simulink library "csu_ctp_coarse_thruster_pulse_command_new_lib"  (R2015b)
settings: Solver=ode113  StartTime=0.0  StopTime=10.0  RelTol=1e-3
values from neighbouring files (symbols this model uses):
  cac_acs_minimum_coarse_thruster_ontime = 30    [csc_cac_coarse_acs_ctrl_init.m]
  cac_acs_time_gain_x = 20.0    (= 20)    [csc_cac_coarse_acs_ctrl_init.m]
  cac_acs_time_gain_y = 20.0    (= 20)    [csc_cac_coarse_acs_ctrl_init.m]
  cac_acs_time_gain_z = 20.0    (= 20)    [csc_cac_coarse_acs_ctrl_init.m]
  cac_coarse_desired_thrust_gain = 1.0    (= 1)    [csc_cac_coarse_acs_ctrl_init.m]
  cac_coarse_thruster_force = psp_coarse_acs_thrust    [csc_cac_coarse_acs_ctrl_prep.m]
  cac_coarse_thruster_trq_x = cac_coarse_thruster_trq_x + cac_coarse_thruster_force*cac_coarse_trq_matx(cac_thruster_alloc_coarse_x_plus(i),1)    [csc_cac_coarse_acs_ctrl_prep.m]
  cac_coarse_thruster_trq_y = cac_coarse_thruster_trq_y + cac_coarse_thruster_force*cac_coarse_trq_matx(cac_thruster_alloc_coarse_y_plus(i),2)    [csc_cac_coarse_acs_ctrl_prep.m]
  cac_coarse_thruster_trq_z = cac_coarse_thruster_trq_z + cac_coarse_thruster_force*cac_coarse_trq_matx(cac_thruster_alloc_coarse_z_plus(i),3)    [csc_cac_coarse_acs_ctrl_prep.m]
  cac_max_thrust_to_weight_ratio = 1.05    [csc_cac_coarse_acs_ctrl_init.m]
  cac_saturation_axial_force = 0*cac_coarse_thruster_force*cosd(15)+4*cac_coarse_thruster_force    [csc_cac_coarse_acs_ctrl_prep.m]
  cac_total_trq_axial_force_matx = [cac_coarse_thruster_force*cac_coarse_trq_matx';cac_coarse_thruster_force_axial]    [csc_cac_coarse_acs_ctrl_prep.m]
undefined symbols (not defined in the file or in its folder): cac_num_variable, cac_thr_control, cac_thruster_alloc_pad_coarse_x_tq_full_on, cac_thruster_alloc_pad_coarse_x_tq_variable, cac_thruster_alloc_pad_coarse_y_tq_full_on, cac_thruster_alloc_pad_coarse_y_tq_variable, cac_trq_control, emp_initial_mass, gal_grav_surface_topo
libraries: simulink x12, util_info_lib x2
(part 1 of 2)
settings Model: Creator=Jim Kaidy  LastModifiedBy=jimkaidy
settings DataIOCC: SaveFormat=Array  SignalLoggingSaveFormat=ModelDataLogs
settings DebuggingCC: AlgebraicLoopMsg=error  ArtificialAlgebraicLoopMsg=error  UnderspecifiedInitializationDetection=Classic  MergeDetectMultiDrivingBlocksExec=none  SolverPrmCheckMsg=warning
settings HardwareCC: ProdBitPerPointer=32  ProdLargestAtomicFloat=None  ProdIntDivRoundTo=Undefined  ProdEndianess=Unspecified  ProdWordSize=32  ProdHWDeviceType=32-bit Generic
settings GRTTargetCC: GeneratePreprocessorConditionals=Disable all
settings ConfigComp: CovModelRefEnable=Off  CovSFcnEnable=off

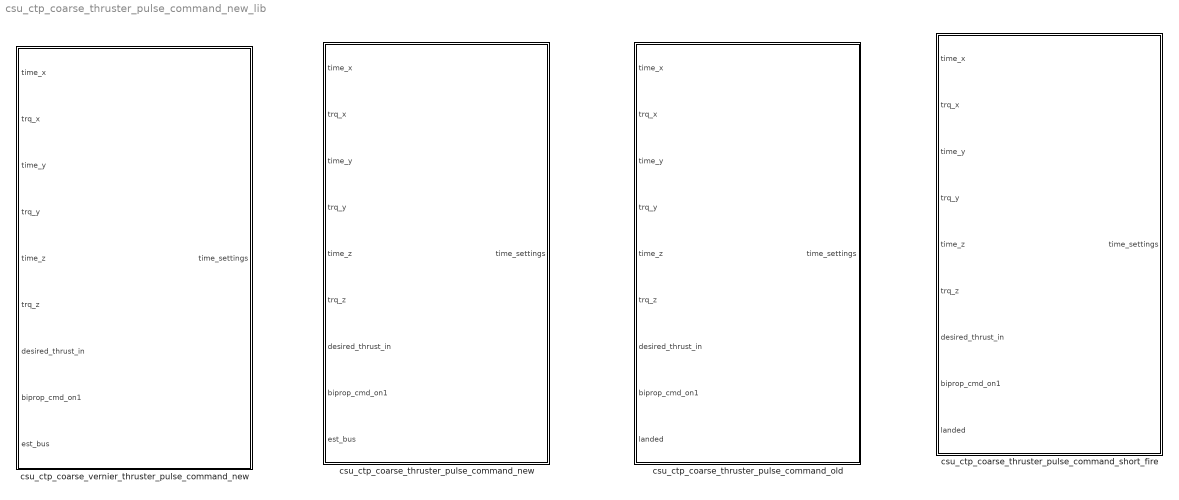
== system csu_ctp_coarse_thruster_pulse_command_new_lib ==
  csu_ctp_coarse_thruster_pulse_command_new : Subsystem
  csu_ctp_coarse_thruster_pulse_command_old : Subsystem
  csu_ctp_coarse_thruster_pulse_command_short_fire : Subsystem
  csu_ctp_coarse_vernier_thruster_pulse_command_new : Subsystem

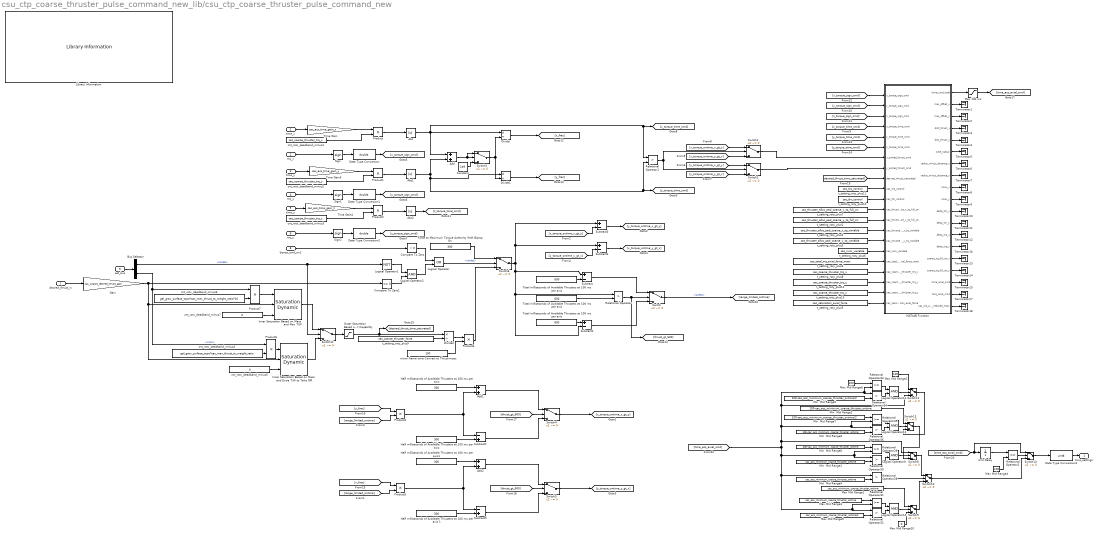
== system csu_ctp_coarse_thruster_pulse_command_new_lib/csu_ctp_coarse_thruster_pulse_command_new ==
  time_x : Inport
  "trq_x " : Inport  Port=2
  time_y : Inport  Port=3
  trq_y : Inport  Port=4
  time_z : Inport  Port=5
  trq_z : Inport  Port=6
  desired_thrust_in : Inport  Port=7
  biprop_cmd_on1 : Inport  Port=8
  est_bus : Inport  Port=9
  Abs : Abs
  Abs1 : Abs
  Abs2 : Abs
  Add : Sum
  Add1 : Sum
  Add2 : Sum
  Bus Selector : BusSelector  OutputSignals=landed,mass
  Compare To Zero : simulink/Logic and Bit Operations/Compare To Zero  relop=>  OutDataTypeStr=boolean
  Compare To Zero1 : simulink/Logic and Bit Operations/Compare To Zero  relop===  OutDataTypeStr=boolean
  Constant : Constant  Value=1e9
  Data Type Conversion : DataTypeConversion  OutDataTypeStr=double
  Data Type Conversion1 : DataTypeConversion  OutDataTypeStr=double
  Data Type Conversion2 : DataTypeConversion  OutDataTypeStr=double
  Data Type Conversion3 : DataTypeConversion  OutDataTypeStr=uint8
  Divide : Product  Inputs=*/
  Divide1 : Product  Inputs=*/
  Divide2 : Product  Inputs=*/
  Force to Maximum Torque Authority With Biprop On : Constant  Value=300
  Gain : Gain  Gain=cac_coarse_desired_thrust_gain
  Half milliseconds of Available Thrusters at 100 ms per axis : Constant  Value=300
  "Half milliseconds of Available Thrusters at 100 ms per axis " : Constant  Value=300
  Half milliseconds of Available Thrusters at 100 ms per axis 1 : Constant  Value=300
  Half milliseconds of Available Thrusters at 100 ms per axis1 : Constant  Value=300
  Inner Saturation Based on Mass and Extra T/W to Take Off : simulink/Discontinuities/Saturation Dynamic  OutMin=[]  OutMax=[]  OutDataTypeStr=Inherit: Same as second input  OutDataType=fixdt(1, 16)  OutScaling=2^-10  DoSatur=off
  Inner Saturation Based on Mass and Max T/W : simulink/Discontinuities/Saturation Dynamic  OutMin=[]  OutMax=[]  OutDataTypeStr=Inherit: Same as second input  OutDataType=fixdt(1, 16)  OutScaling=2^-10  DoSatur=off
  Library Information : util_info_lib/Library Information  owner='NONE'
  Logical Operator : Logic  Operator=OR  AllPortsSameDT=off  OutDataTypeStr=boolean
  Logical Operator1 : Logic  Operator=NOT  AllPortsSameDT=off  OutDataTypeStr=boolean
  Logical Operator{2,9..12} (5 alike) : Logic  AllPortsSameDT=off  OutDataTypeStr=boolean
  MATLAB Function : MATLAB Function  TreatAsAtomicUnit=on
  Max 100 ms : Saturate  UpperLimit=100  LowerLimit=0
  Max Mid Range1 : Constant  Value=cac_acs_minimum_coarse_thruster_ontime
  Max Mid Range10 : Constant  Value=0
  Max Mid Range2 : Constant  Value=100
  Max Mid Range3 : Constant  Value=cac_acs_minimum_coarse_thruster_ontime
  Max Mid Range4 : Constant  Value=100
  Max Mid Range6 : Constant  Value=100
  Max Mid Range9 : Constant  Value=cac_acs_minimum_coarse_thruster_ontime/2
  Min  Mid Range1 : Constant  Value=cac_acs_minimum_coarse_thruster_ontime
  Min  Mid Range2 : Constant  Value=100-cac_acs_minimum_coarse_thruster_ontime
  Min  Mid Range4 : Constant  Value=cac_acs_minimum_coarse_thruster_ontime
  Min  Mid Range5 : Constant  Value=100-cac_acs_minimum_coarse_thruster_ontime/2
  Min  Mid Range6 : Constant  Value=100-cac_acs_minimum_coarse_thruster_ontime
  Min  Mid Range7 : Constant  Value=100-cac_acs_minimum_coarse_thruster_ontime/2
  Min  Mid Range8 : Constant  Value=100-cac_acs_minimum_coarse_thruster_ontime
  Outer Saturation Based on Total Thrust Capability : Saturate  UpperLimit=cac_saturation_axial_force  LowerLimit=0
  Product{,1..7} (8 alike) : Product
  Relational Operator{,1,28,30,32,34,36} (7 alike) : RelationalOperator  Operator=>  OutDataTypeStr=boolean
  Relational Operator2 : RelationalOperator  Operator===  OutDataTypeStr=boolean
  Relational Operator{29,31,33,35} (4 alike) : RelationalOperator  OutDataTypeStr=boolean
  Sign : Signum
  Sign1 : Signum
  Sign2 : Signum
  Subtract{,2..4} (4 alike) : Sum  Inputs=+-
  Subtract1 : Sum  Inputs=-+
  Subtract5 : Sum  Inputs=-+
  Switch{,1..6,8..14} (14 alike) : Switch  Criteria=u2 ~= 0
  Terminator{1..18} (18 alike) : Terminator
  Time Gain : Gain  Gain=cac_acs_time_gain_x
  Time Gain3 : Gain  Gain=cac_acs_time_gain_y
  Time Gain4 : Gain  Gain=cac_acs_time_gain_z
  Total milliseconds of Available Thrusters at 100 ms per axis : Constant  Value=600
  "Total milliseconds of Available Thrusters at 100 ms per axis " : Constant  Value=600
  "Total milliseconds of Available Thrusters at 100 ms per axis  " : Constant  Value=600
  Unit Delay : UnitDelay  SampleTime=-1
  cnt_rotx_deadband_minus1 : Constant  Value=cac_coarse_thruster_trq_x
  cnt_rotx_deadband_minus2 : Constant  Value=cac_coarse_thruster_trq_y
  cnt_rotx_deadband_minus3 : Constant  Value=cac_coarse_thruster_trq_z
  cnt_rotx_deadband_minus4 : Constant  Value=gal_grav_surface_topo*cac_max_thrust_to_weight_ratio
  cnt_rotx_deadband_minus5 : Constant  Value=0
  cnt_rotx_deadband_minus6 : Constant  Value=gal_grav_surface_topo*cac_max_thrust_to_weight_ratio*10
  cnt_rotx_deadband_minus7 : Constant  Value=0
  "minor frame time Convert to Thrust-msec " : Constant  Value=100
  t_setting_roty_plus1 : Constant  Value=cac_thruster_alloc_pad_coarse_y_tq_full_on
  t_setting_roty_plus10 : Constant  Value=cac_thr_control
  t_setting_roty_plus11 : Constant  Value=cac_trq_control
  t_setting_roty_plus12 : Constant  Value=cac_coarse_thruster_trq_y
  t_setting_roty_plus13 : Constant  Value=cac_coarse_thruster_trq_z
  t_setting_roty_plus2 : Constant  Value=cac_thruster_alloc_pad_coarse_x_tq_variable
  t_setting_roty_plus3 : Constant  Value=cac_thruster_alloc_pad_coarse_y_tq_variable
  t_setting_roty_plus4 : Constant  Value=cac_total_trq_axial_force_matx
  t_setting_roty_plus5 : Constant  Value=cac_saturation_axial_force
  t_setting_roty_plus6 : Constant  Value=cac_num_variable
  t_setting_roty_plus7 : Constant  Value=cac_thruster_alloc_pad_coarse_x_tq_full_on
  t_setting_roty_plus8 : Constant  Value=cac_coarse_thruster_trq_x
  t_setting_roty_plus9 : Constant  Value=cac_coarse_thruster_force
  time_settings : Outport
  wires:
  Bus Selector/2 -> Product7/1, Product6/1  "<mass>"
  Product7/1 -> Inner Saturation Based on Mass and Max T/W/1
  cnt_rotx_deadband_minus6/1 -> Product7/2
  cnt_rotx_deadband_minus7/1 -> Inner Saturation Based on Mass and Max T/W/3
  Product6/1 -> Inner Saturation Based on Mass and Extra T/W to Take Off/1
  cnt_rotx_deadband_minus4/1 -> Product6/2
  cnt_rotx_deadband_minus5/1 -> Inner Saturation Based on Mass and Extra T/W to Take Off/3
  est_bus/1 -> Bus Selector/1
  Data Type Conversion3/1 -> time_settings/1
  Min  Mid Range6/1 -> Relational Operator29/1
  Min  Mid Range1/1 -> Relational Operator30/2
  Relational Operator29/1 -> Logical Operator9/1
  Relational Operator30/1 -> Logical Operator9/2
  Max Mid Range3/1 -> Relational Operator31/1
  Max Mid Range9/1 -> Relational Operator32/2
  Relational Operator31/1 -> Logical Operator10/1
  Relational Operator32/1 -> Logical Operator10/2
  Logical Operator10/1 -> Switch9/2
  Max Mid Range1/1 -> Switch9/1
  Logical Operator9/1 -> Switch8/2
  Switch9/1 -> Switch10/3
  Switch14/1 -> Data Type Conversion3/1
  Min  Mid Range4/1 -> Relational Operator28/2
  Relational Operator28/1 -> Switch10/2
  Switch8/1 -> Switch10/1
  Max Mid Range6/1 -> Relational Operator33/1
  Min  Mid Range5/1 -> Relational Operator34/2
  Min  Mid Range7/1 -> Relational Operator35/1
  Min  Mid Range8/1 -> Relational Operator36/2
  Relational Operator33/1 -> Logical Operator11/1
  Relational Operator34/1 -> Logical Operator11/2
  Logical Operator11/1 -> Switch12/2
  Max Mid Range2/1 -> Switch12/1
  Relational Operator35/1 -> Logical Operator12/1
  Relational Operator36/1 -> Logical Operator12/2
  Logical Operator12/1 -> Switch13/2
  Min  Mid Range2/1 -> Switch13/1
  Switch13/1 -> Switch8/3
  Switch12/1 -> Switch13/3
  Max Mid Range10/1 -> Switch9/3
  cnt_rotx_deadband_minus1/1 -> Product/2
  time_x/1 -> Time Gain/1
  time_y/1 -> Time Gain3/1
  time_z/1 -> Time Gain4/1
  cnt_rotx_deadband_minus2/1 -> Product1/2
  cnt_rotx_deadband_minus3/1 -> Product2/2
  Product/1 -> Abs/1
  Product1/1 -> Abs1/1
  "minor frame time Convert to Thrust-msec "/1 -> Product3/2
  t_setting_roty_plus9/1 -> Divide2/2
  Divide2/1 -> Product3/1
  Total milliseconds of Available Thrusters at 100 ms per axis/1 -> Relational Operator/2
  Relational Operator/1 -> [thrust_gt_600], Switch/2
  "Total milliseconds of Available Thrusters at 100 ms per axis "/1 -> Subtract/2
  Subtract/1 -> Switch/1
  "Total milliseconds of Available Thrusters at 100 ms per axis  "/1 -> Subtract2/1
  Subtract2/1 -> Switch/3
  Divide1/1 -> [y_frac]
  [x_torque_ontime_x_gt_y] -> Subtract3/2
  Subtract3/1 -> [y_torque_ontime_x_gt_y]
  [y_torque_ontime_y_gt_x] -> Subtract4/2
  Subtract4/1 -> [x_torque_ontime_y_gt_x]
  Relational Operator1/1 -> Switch1/2, Switch2/2
  [y_torque_ontime_x_gt_y] -> Switch2/1
  [y_torque_ontime_y_gt_x] -> Switch2/3
  [x_torque_ontime_y_gt_x] -> Switch1/3
  [x_torque_ontime_x_gt_y] -> Switch1/1
  Sign/1 -> Data Type Conversion/1
  "trq_x "/1 -> Sign/1
  Sign1/1 -> Data Type Conversion1/1
  trq_y/1 -> Sign1/1
  Sign2/1 -> Data Type Conversion2/1
  trq_z/1 -> Sign2/1
  Data Type Conversion2/1 -> [z_torque_sign_cmd]
  Data Type Conversion1/1 -> [y_torque_sign_cmd]
  Data Type Conversion/1 -> [x_torque_sign_cmd]
  [y_torque_time_cmd] -> MATLAB Function/5(y_torque_time_cmd)
  [x_torque_time_cmd] -> MATLAB Function/4(x_torque_time_cmd)
  [y_torque_sign_cmd] -> MATLAB Function/2(y_torque_sign_cmd)
  Switch2/1 -> MATLAB Function/8(y_sorted_thrust_cmd)
  Product2/1 -> Abs2/1
  Abs2/1 -> [z_torque_time_cmd]
  [x_torque_sign_cmd] -> MATLAB Function/1(x_torque_sign_cmd)
  Switch6/1 -> Subtract3/1, Subtract4/1, Subtract2/2, Relational Operator/1, Subtract/1
  Add/1 -> Switch3/1, Switch3/2
  Constant/1 -> Switch3/3
  Switch3/1 -> Divide1/2, Divide/2
  Divide/1 -> [x_frac]
  MATLAB Function/1(time_cmd_total) -> Max 100 ms/1
  [z_torque_sign_cmd] -> MATLAB Function/3(z_torque_sign_cmd)
  [z_torque_time_cmd] -> MATLAB Function/6(z_torque_time_cmd)
  t_setting_roty_plus1/1 -> MATLAB Function/13(cac_thruster_alloc_pad_coarse_y_tq_full_on)
  t_setting_roty_plus11/1 -> MATLAB Function/10(cac_trq_control)
  t_setting_roty_plus8/1 -> MATLAB Function/18(cac_coarse_thruster_trq_x)
  t_setting_roty_plus2/1 -> MATLAB Function/14(cac_thruster_alloc_pad_coarse_x_tq_variable)
  t_setting_roty_plus13/1 -> MATLAB Function/20(cac_coarse_thruster_trq_z)
  t_setting_roty_plus5/1 -> MATLAB Function/21(cac_saturation_axial_force)
  t_setting_roty_plus6/1 -> MATLAB Function/16(cac_num_variable)
  t_setting_roty_plus10/1 -> MATLAB Function/11(cac_thr_control)
  t_setting_roty_plus7/1 -> MATLAB Function/12(cac_thruster_alloc_pad_coarse_x_tq_full_on)
  t_setting_roty_plus12/1 -> MATLAB Function/19(cac_coarse_thruster_trq_y)
  t_setting_roty_plus4/1 -> MATLAB Function/17(cac_total_trq_axial_force_matx)
  t_setting_roty_plus3/1 -> MATLAB Function/15(cac_thruster_alloc_pad_coarse_y_tq_variable)
  Time Gain/1 -> Product/1
  Time Gain4/1 -> Product2/1
  "Half milliseconds of Available Thrusters at 100 ms per axis "/1 -> Subtract1/2
  Product4/1 -> Subtract1/1, Add1/2
  Half milliseconds of Available Thrusters at 100 ms per axis/1 -> Add1/1
  [x_frac] -> Product5/1
  [range_limited_ontime] -> Product5/2
  [y_frac] -> Product4/1
  [range_limited_ontime] -> Product4/2
  [thrust_gt_600] -> Switch4/2
  Add1/1 -> Switch4/1
  Subtract1/1 -> Switch4/3
  Half milliseconds of Available Thrusters at 100 ms per axis 1/1 -> Subtract5/2
  Product5/1 -> Add2/2, Subtract5/1
  Half milliseconds of Available Thrusters at 100 ms per axis1/1 -> Add2/1
  [thrust_gt_600] -> Switch5/2
  Add2/1 -> Switch5/1
  Subtract5/1 -> Switch5/3
  Switch4/1 -> [x_torque_ontime_x_gt_y]
  Switch5/1 -> [y_torque_ontime_y_gt_x]
  [time_acs_axial_cmd] -> Relational Operator32/1, Relational Operator31/2, Relational Operator28/1, Relational Operator29/2, Relational Operator30/1, Relational Operator34/1, Relational Operator33/2, Switch12/3, Relational Operator35/2, Relational Operator36/1, Switch8/1
  [desired_thrust_time_saturated] -> MATLAB Function/9(desired_thrust_saturated)
  Time Gain3/1 -> Product1/1
  Max 100 ms/1 -> [time_acs_axial_cmd]
  biprop_cmd_on1/1 -> Compare To Zero/1
  Outer Saturation Based on Total Thrust Capability/1 -> [desired_thrust_time_saturated], Divide2/1
  Force to Maximum Torque Authority With Biprop On/1 -> Switch6/1
  Compare To Zero/1 -> Logical Operator/1
  Logical Operator1/1 -> Logical Operator2/1
  Compare To Zero1/1 -> Logical Operator2/2
  Logical Operator2/1 -> Logical Operator/2
  Bus Selector/1 -> Logical Operator1/1, Switch11/2  "<landed>"
  Switch11/1 -> Outer Saturation Based on Total Thrust Capability/1
  Inner Saturation Based on Mass and Extra T/W to Take Off/1 -> Switch11/3
  desired_thrust_in/1 -> Gain/1
  MATLAB Function/2(max_offset_x) -> Terminator1/1
  MATLAB Function/19(cac_trq_axial_force_pinv_reduced_matx) -> Terminator18/1
  MATLAB Function/16(coarse_tq_full_on_y) -> Terminator14/1
  MATLAB Function/11(delta_thr_x) -> Terminator10/1
  MATLAB Function/15(coarse_tq_full_on_x) -> Terminator13/1
  MATLAB Function/3(max_offset_y) -> Terminator2/1
  MATLAB Function/13(delta_trq_x) -> Terminator12/1
  Switch1/1 -> MATLAB Function/7(x_sorted_thrust_cmd)
  Abs/1 -> Relational Operator1/1, [x_torque_time_cmd], Add/1, Divide/1
  Abs1/1 -> Divide1/1, [y_torque_time_cmd], Relational Operator1/2, Add/2
  Gain/1 -> Compare To Zero1/1, Inner Saturation Based on Mass and Max T/W/2, Inner Saturation Based on Mass and Extra T/W to Take Off/2
  MATLAB Function/12(delta_thr_y) -> Terminator11/1
  MATLAB Function/14(delta_trq_y) -> Terminator16/1
  Inner Saturation Based on Mass and Max T/W/1 -> Switch11/1
  Logical Operator/1 -> Switch6/2  "<landed>"
  Switch/1 -> [range_limited_ontime]  "<landed>"
  Product3/1 -> Switch6/3
  MATLAB Function/10(imax_y) -> Terminator9/1
  MATLAB Function/4(dist_thrust_x) -> Terminator3/1
  MATLAB Function/5(dist_thrust_y) -> Terminator4/1
  MATLAB Function/6(zone_radius) -> Terminator5/1
  MATLAB Function/7(radius_minus_distance_x) -> Terminator6/1
  MATLAB Function/8(radius_minus_distance_y) -> Terminator7/1
  MATLAB Function/9(imax_x) -> Terminator8/1
  MATLAB Function/18(torq_axial_cmd) -> Terminator17/1
  MATLAB Function/17(time_axial_cmd) -> Terminator15/1
  Switch10/1 -> Switch14/3
  Unit Delay/1 -> Relational Operator2/1
  Max Mid Range4/1 -> Relational Operator2/2
  Relational Operator2/1 -> Switch14/2
  [time_acs_axial_cmd] -> Switch14/1, Unit Delay/1

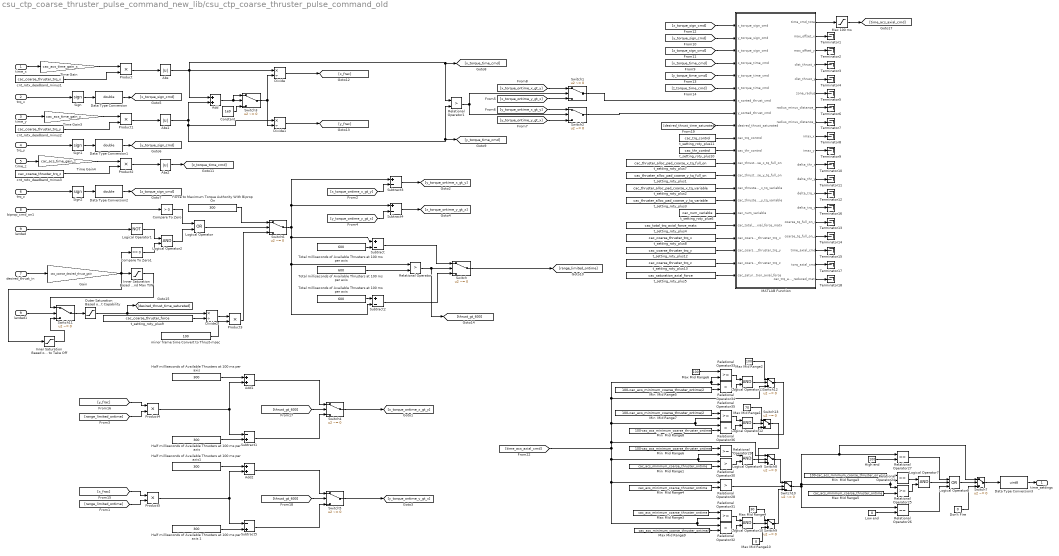
== system csu_ctp_coarse_thruster_pulse_command_new_lib/csu_ctp_coarse_thruster_pulse_command_old ==
  time_x : Inport
  "trq_x " : Inport  Port=2
  time_y : Inport  Port=3
  trq_y : Inport  Port=4
  time_z : Inport  Port=5
  trq_z : Inport  Port=6
  desired_thrust_in : Inport  Port=7
  biprop_cmd_on1 : Inport  Port=8
  landed : Inport  Port=9
  Abs : Abs
  Abs1 : Abs
  Abs2 : Abs
  Add : Sum
  Add1 : Sum
  Add2 : Sum
  Compare To Zero : simulink/Logic and Bit Operations/Compare To Zero  relop=>  OutDataTypeStr=boolean
  Compare To Zero1 : simulink/Logic and Bit Operations/Compare To Zero  relop===  OutDataTypeStr=boolean
  Constant : Constant  Value=1e9
  Data Type Conversion : DataTypeConversion  OutDataTypeStr=double
  Data Type Conversion1 : DataTypeConversion  OutDataTypeStr=double
  Data Type Conversion2 : DataTypeConversion  OutDataTypeStr=double
  Data Type Conversion3 : DataTypeConversion  OutDataTypeStr=uint8
  Divide : Product  Inputs=*/
  Divide1 : Product  Inputs=*/
  Divide2 : Product  Inputs=*/
  Don't Fire : Constant  Value=0
  Force to Maximum Torque Authority With Biprop On : Constant  Value=300
  Gain : Gain  Gain=cac_coarse_desired_thrust_gain
  Half milliseconds of Available Thrusters at 100 ms per axis : Constant  Value=300
  "Half milliseconds of Available Thrusters at 100 ms per axis " : Constant  Value=300
  Half milliseconds of Available Thrusters at 100 ms per axis 1 : Constant  Value=300
  Half milliseconds of Available Thrusters at 100 ms per axis1 : Constant  Value=300
  High end : Constant  Value=100
  Inner Saturation Based on Mass and Extra T/W to Take Off : Saturate  UpperLimit=emp_initial_mass*gal_grav_surface_topo*cac_max_thrust_to_weight_ratio*10  LowerLimit=0
  Inner Saturation Based on Mass and Max T/W : Saturate  UpperLimit=emp_initial_mass*gal_grav_surface_topo*cac_max_thrust_to_weight_ratio  LowerLimit=0
  Logical Operator : Logic  Operator=OR  AllPortsSameDT=off  OutDataTypeStr=boolean
  Logical Operator1 : Logic  Operator=NOT  AllPortsSameDT=off  OutDataTypeStr=boolean
  Logical Operator{2,7,9..12} (6 alike) : Logic  AllPortsSameDT=off  OutDataTypeStr=boolean
  Logical Operator8 : Logic  Operator=OR  Inputs=3  AllPortsSameDT=off  OutDataTypeStr=boolean
  Low end : Constant  Value=0
  MATLAB Function : MATLAB Function  TreatAsAtomicUnit=on
  Max 100 ms : Saturate  UpperLimit=100  LowerLimit=0
  Max Mid Range1 : Constant  Value=70
  Max Mid Range10 : Constant  Value=0
  Max Mid Range2 : Constant  Value=100
  Max Mid Range3 : Constant  Value=cac_acs_minimum_coarse_thruster_ontime
  Max Mid Range4 : Constant  Value=30
  Max Mid Range5 : Constant  Value=cac_acs_minimum_coarse_thruster_ontime
  Max Mid Range6 : Constant  Value=100
  Max Mid Range9 : Constant  Value=cac_acs_minimum_coarse_thruster_ontime/2
  Min  Mid Range1 : Constant  Value=cac_acs_minimum_coarse_thruster_ontime
  Min  Mid Range3 : Constant  Value=100-cac_acs_minimum_coarse_thruster_ontime
  Min  Mid Range4 : Constant  Value=cac_acs_minimum_coarse_thruster_ontime
  Min  Mid Range5 : Constant  Value=100-cac_acs_minimum_coarse_thruster_ontime/2
  Min  Mid Range6 : Constant  Value=100-cac_acs_minimum_coarse_thruster_ontime
  Min  Mid Range7 : Constant  Value=100-cac_acs_minimum_coarse_thruster_ontime/2
  Min  Mid Range8 : Constant  Value=100-cac_acs_minimum_coarse_thruster_ontime
  Outer Saturation Based on Total Thrust Capability : Saturate  UpperLimit=cac_saturation_axial_force  LowerLimit=0
  Product{,1..5} (6 alike) : Product
  Relational Operator{,1,28,30,32,34,36} (7 alike) : RelationalOperator  Operator=>  OutDataTypeStr=boolean
  Relational Operator{24..25,29,31,33,35} (6 alike) : RelationalOperator  OutDataTypeStr=boolean
  Relational Operator26 : RelationalOperator  Operator===  OutDataTypeStr=boolean
  Relational Operator27 : RelationalOperator  Operator===  OutDataTypeStr=boolean
  Sign : Signum
  Sign1 : Signum
  Sign2 : Signum
  Subtract{,2..4} (4 alike) : Sum  Inputs=+-
  Subtract1 : Sum  Inputs=-+
  Subtract5 : Sum  Inputs=-+
  Switch{,1..13} (14 alike) : Switch  Criteria=u2 ~= 0
  Terminator{1..18} (18 alike) : Terminator
  Time Gain : Gain  Gain=cac_acs_time_gain_x
  Time Gain3 : Gain  Gain=cac_acs_time_gain_y
  Time Gain4 : Gain  Gain=cac_acs_time_gain_z
  Total milliseconds of Available Thrusters at 100 ms per axis : Constant  Value=600
  "Total milliseconds of Available Thrusters at 100 ms per axis " : Constant  Value=600
  "Total milliseconds of Available Thrusters at 100 ms per axis  " : Constant  Value=600
  cnt_rotx_deadband_minus1 : Constant  Value=cac_coarse_thruster_trq_x
  cnt_rotx_deadband_minus2 : Constant  Value=cac_coarse_thruster_trq_y
  cnt_rotx_deadband_minus3 : Constant  Value=cac_coarse_thruster_trq_z
  landed1 : InportShadow  Port=9
  "minor frame time Convert to Thrust-msec " : Constant  Value=100
  t_setting_roty_plus1 : Constant  Value=cac_thruster_alloc_pad_coarse_y_tq_full_on
  t_setting_roty_plus10 : Constant  Value=cac_thr_control
  t_setting_roty_plus11 : Constant  Value=cac_trq_control
  t_setting_roty_plus12 : Constant  Value=cac_coarse_thruster_trq_y
  t_setting_roty_plus13 : Constant  Value=cac_coarse_thruster_trq_z
  t_setting_roty_plus2 : Constant  Value=cac_thruster_alloc_pad_coarse_x_tq_variable
  t_setting_roty_plus3 : Constant  Value=cac_thruster_alloc_pad_coarse_y_tq_variable
  t_setting_roty_plus4 : Constant  Value=cac_total_trq_axial_force_matx
  t_setting_roty_plus5 : Constant  Value=cac_saturation_axial_force
  t_setting_roty_plus6 : Constant  Value=cac_num_variable
  t_setting_roty_plus7 : Constant  Value=cac_thruster_alloc_pad_coarse_x_tq_full_on
  t_setting_roty_plus8 : Constant  Value=cac_coarse_thruster_trq_x
  t_setting_roty_plus9 : Constant  Value=cac_coarse_thruster_force
  time_settings : Outport
  wires:
  Data Type Conversion3/1 -> time_settings/1
  Relational Operator24/1 -> Logical Operator7/1
  Relational Operator25/1 -> Logical Operator7/2
  Min  Mid Range3/1 -> Relational Operator24/1
  Max Mid Range5/1 -> Relational Operator25/2
  High end/1 -> Relational Operator27/2
  Relational Operator27/1 -> Logical Operator8/1
  Logical Operator7/1 -> Logical Operator8/2
  Relational Operator26/1 -> Logical Operator8/3
  Low end/1 -> Relational Operator26/2
  Logical Operator8/1 -> Switch7/2
  Don't Fire/1 -> Switch7/3
  Min  Mid Range6/1 -> Relational Operator29/1
  Min  Mid Range1/1 -> Relational Operator30/2
  Relational Operator29/1 -> Logical Operator9/1
  Relational Operator30/1 -> Logical Operator9/2
  Max Mid Range3/1 -> Relational Operator31/1
  Max Mid Range9/1 -> Relational Operator32/2
  Relational Operator31/1 -> Logical Operator10/1
  Relational Operator32/1 -> Logical Operator10/2
  Logical Operator10/1 -> Switch9/2
  Max Mid Range4/1 -> Switch9/1
  Logical Operator9/1 -> Switch8/2
  Switch9/1 -> Switch10/3
  Switch10/1 -> Relational Operator25/1, Relational Operator24/2, Switch7/1, Relational Operator27/1, Relational Operator26/1
  Min  Mid Range4/1 -> Relational Operator28/2
  Relational Operator28/1 -> Switch10/2
  Switch8/1 -> Switch10/1
  Max Mid Range6/1 -> Relational Operator33/1
  Min  Mid Range5/1 -> Relational Operator34/2
  Min  Mid Range7/1 -> Relational Operator35/1
  Min  Mid Range8/1 -> Relational Operator36/2
  Relational Operator33/1 -> Logical Operator11/1
  Relational Operator34/1 -> Logical Operator11/2
  Logical Operator11/1 -> Switch12/2
  Max Mid Range2/1 -> Switch12/1
  Relational Operator35/1 -> Logical Operator12/1
  Relational Operator36/1 -> Logical Operator12/2
  Logical Operator12/1 -> Switch13/2
  Max Mid Range1/1 -> Switch13/1
  Switch13/1 -> Switch8/3
  Switch12/1 -> Switch13/3
  Max Mid Range10/1 -> Switch9/3
  cnt_rotx_deadband_minus1/1 -> Product/2
  time_x/1 -> Time Gain/1
  time_y/1 -> Time Gain3/1
  time_z/1 -> Time Gain4/1
  cnt_rotx_deadband_minus2/1 -> Product1/2
  cnt_rotx_deadband_minus3/1 -> Product2/2
  Product/1 -> Abs/1
  Product1/1 -> Abs1/1
  "minor frame time Convert to Thrust-msec "/1 -> Product3/2
  t_setting_roty_plus9/1 -> Divide2/2
  Divide2/1 -> Product3/1
  Total milliseconds of Available Thrusters at 100 ms per axis/1 -> Relational Operator/2
  Relational Operator/1 -> [thrust_gt_600], Switch/2
  "Total milliseconds of Available Thrusters at 100 ms per axis "/1 -> Subtract/2
  Subtract/1 -> Switch/1
  "Total milliseconds of Available Thrusters at 100 ms per axis  "/1 -> Subtract2/1
  Subtract2/1 -> Switch/3
  Divide1/1 -> [y_frac]
  [x_torque_ontime_x_gt_y] -> Subtract3/2
  Subtract3/1 -> [y_torque_ontime_x_gt_y]
  [y_torque_ontime_y_gt_x] -> Subtract4/2
  Subtract4/1 -> [x_torque_ontime_y_gt_x]
  Relational Operator1/1 -> Switch1/2, Switch2/2
  [y_torque_ontime_x_gt_y] -> Switch2/1
  [y_torque_ontime_y_gt_x] -> Switch2/3
  [x_torque_ontime_y_gt_x] -> Switch1/3
  [x_torque_ontime_x_gt_y] -> Switch1/1
  Sign/1 -> Data Type Conversion/1
  "trq_x "/1 -> Sign/1
  Sign1/1 -> Data Type Conversion1/1
  trq_y/1 -> Sign1/1
  Sign2/1 -> Data Type Conversion2/1
  trq_z/1 -> Sign2/1
  Data Type Conversion2/1 -> [z_torque_sign_cmd]
  Data Type Conversion1/1 -> [y_torque_sign_cmd]
  Data Type Conversion/1 -> [x_torque_sign_cmd]
  [y_torque_time_cmd] -> MATLAB Function/5(y_torque_time_cmd)
  [x_torque_time_cmd] -> MATLAB Function/4(x_torque_time_cmd)
  [y_torque_sign_cmd] -> MATLAB Function/2(y_torque_sign_cmd)
  Switch2/1 -> MATLAB Function/8(y_sorted_thrust_cmd)
  Product2/1 -> Abs2/1
  Abs2/1 -> [z_torque_time_cmd]
  [x_torque_sign_cmd] -> MATLAB Function/1(x_torque_sign_cmd)
  Switch6/1 -> Subtract3/1, Subtract4/1, Subtract2/2, Relational Operator/1, Subtract/1
  Add/1 -> Switch3/1, Switch3/2
  Constant/1 -> Switch3/3
  Switch3/1 -> Divide1/2, Divide/2
  Divide/1 -> [x_frac]
  MATLAB Function/1(time_cmd_total) -> Max 100 ms/1
  [z_torque_sign_cmd] -> MATLAB Function/3(z_torque_sign_cmd)
  [z_torque_time_cmd] -> MATLAB Function/6(z_torque_time_cmd)
  t_setting_roty_plus1/1 -> MATLAB Function/13(cac_thruster_alloc_pad_coarse_y_tq_full_on)
  t_setting_roty_plus11/1 -> MATLAB Function/10(cac_trq_control)
  t_setting_roty_plus8/1 -> MATLAB Function/18(cac_coarse_thruster_trq_x)
  t_setting_roty_plus2/1 -> MATLAB Function/14(cac_thruster_alloc_pad_coarse_x_tq_variable)
  t_setting_roty_plus13/1 -> MATLAB Function/20(cac_coarse_thruster_trq_z)
  t_setting_roty_plus5/1 -> MATLAB Function/21(cac_saturation_axial_force)
  t_setting_roty_plus6/1 -> MATLAB Function/16(cac_num_variable)
  t_setting_roty_plus10/1 -> MATLAB Function/11(cac_thr_control)
  t_setting_roty_plus7/1 -> MATLAB Function/12(cac_thruster_alloc_pad_coarse_x_tq_full_on)
  t_setting_roty_plus12/1 -> MATLAB Function/19(cac_coarse_thruster_trq_y)
  t_setting_roty_plus4/1 -> MATLAB Function/17(cac_total_trq_axial_force_matx)
  t_setting_roty_plus3/1 -> MATLAB Function/15(cac_thruster_alloc_pad_coarse_y_tq_variable)
  Time Gain/1 -> Product/1
  Time Gain4/1 -> Product2/1
  "Half milliseconds of Available Thrusters at 100 ms per axis "/1 -> Subtract1/2
  Product4/1 -> Subtract1/1, Add1/2
  Half milliseconds of Available Thrusters at 100 ms per axis/1 -> Add1/1
  [x_frac] -> Product5/1
  [range_limited_ontime] -> Product5/2
  [y_frac] -> Product4/1
  [range_limited_ontime] -> Product4/2
  [thrust_gt_600] -> Switch4/2
  Add1/1 -> Switch4/1
  Subtract1/1 -> Switch4/3
  Half milliseconds of Available Thrusters at 100 ms per axis 1/1 -> Subtract5/2
  Product5/1 -> Add2/2, Subtract5/1
  Half milliseconds of Available Thrusters at 100 ms per axis1/1 -> Add2/1
  [thrust_gt_600] -> Switch5/2
  Add2/1 -> Switch5/1
  Subtract5/1 -> Switch5/3
  Switch4/1 -> [x_torque_ontime_x_gt_y]
  Switch5/1 -> [y_torque_ontime_y_gt_x]
  Switch7/1 -> Data Type Conversion3/1
  [time_acs_axial_cmd] -> Relational Operator32/1, Relational Operator31/2, Relational Operator28/1, Relational Operator29/2, Relational Operator30/1, Relational Operator34/1, Relational Operator33/2, Switch12/3, Relational Operator35/2, Relational Operator36/1, Switch8/1
  [desired_thrust_time_saturated] -> MATLAB Function/9(desired_thrust_saturated)
  Time Gain3/1 -> Product1/1
  Max 100 ms/1 -> [time_acs_axial_cmd]
  biprop_cmd_on1/1 -> Compare To Zero/1
  Outer Saturation Based on Total Thrust Capability/1 -> [desired_thrust_time_saturated], Divide2/1
  Force to Maximum Torque Authority With Biprop On/1 -> Switch6/1
  Product3/1 -> Switch6/3
  Compare To Zero/1 -> Logical Operator/1
  Logical Operator/1 -> Switch6/2
  Logical Operator1/1 -> Logical Operator2/1
  Compare To Zero1/1 -> Logical Operator2/2
  Logical Operator2/1 -> Logical Operator/2
  landed/1 -> Logical Operator1/1
  Switch/1 -> [range_limited_ontime]
  Switch11/1 -> Outer Saturation Based on Total Thrust Capability/1
  Inner Saturation Based on Mass and Max T/W/1 -> Switch11/1
  Inner Saturation Based on Mass and Extra T/W to Take Off/1 -> Switch11/3
  landed1/1 -> Switch11/2
  desired_thrust_in/1 -> Gain/1
  MATLAB Function/2(max_offset_x) -> Terminator1/1
  MATLAB Function/19(cac_trq_axial_force_pinv_reduced_matx) -> Terminator18/1
  MATLAB Function/16(coarse_tq_full_on_y) -> Terminator14/1
  MATLAB Function/11(delta_thr_x) -> Terminator10/1
  MATLAB Function/15(coarse_tq_full_on_x) -> Terminator13/1
  MATLAB Function/8(radius_minus_distance_y) -> Terminator7/1
  MATLAB Function/6(zone_radius) -> Terminator5/1
  MATLAB Function/9(imax_x) -> Terminator8/1
  MATLAB Function/7(radius_minus_distance_x) -> Terminator6/1
  MATLAB Function/4(dist_thrust_x) -> Terminator3/1
  MATLAB Function/3(max_offset_y) -> Terminator2/1
  MATLAB Function/5(dist_thrust_y) -> Terminator4/1
  MATLAB Function/17(time_axial_cmd) -> Terminator15/1
  MATLAB Function/13(delta_trq_x) -> Terminator12/1
  Switch1/1 -> MATLAB Function/7(x_sorted_thrust_cmd)
  Abs/1 -> Relational Operator1/1, [x_torque_time_cmd], Add/1, Divide/1
  Abs1/1 -> Divide1/1, [y_torque_time_cmd], Relational Operator1/2, Add/2
  Gain/1 -> Inner Saturation Based on Mass and Extra T/W to Take Off/1, Compare To Zero1/1, Inner Saturation Based on Mass and Max T/W/1
  MATLAB Function/10(imax_y) -> Terminator9/1
  MATLAB Function/12(delta_thr_y) -> Terminator11/1
  MATLAB Function/14(delta_trq_y) -> Terminator16/1
  MATLAB Function/18(torq_axial_cmd) -> Terminator17/1

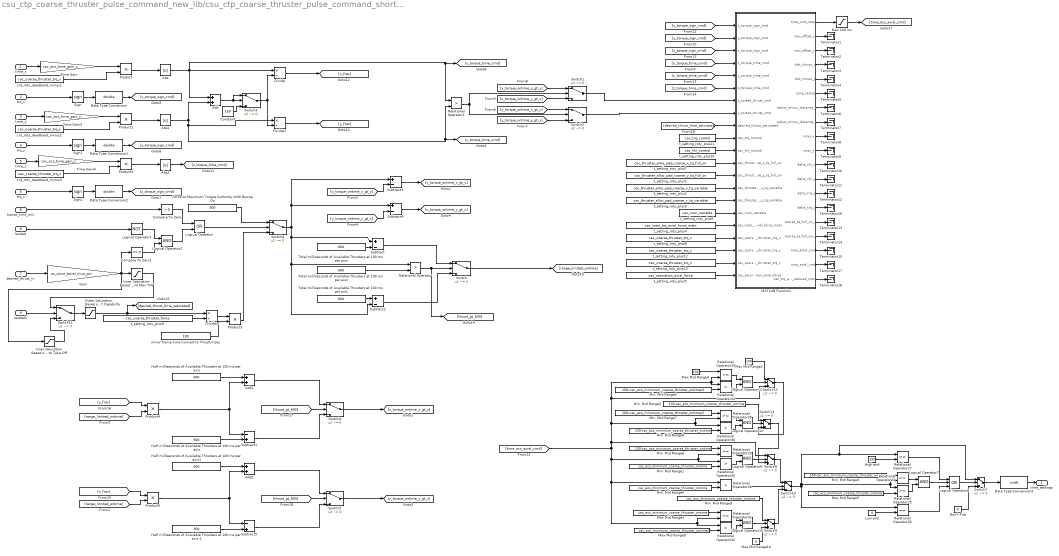
== system csu_ctp_coarse_thruster_pulse_command_new_lib/csu_ctp_coarse_thruster_pulse_command_short_fire ==
  time_x : Inport
  "trq_x " : Inport  Port=2
  time_y : Inport  Port=3
  trq_y : Inport  Port=4
  time_z : Inport  Port=5
  trq_z : Inport  Port=6
  desired_thrust_in : Inport  Port=7
  biprop_cmd_on1 : Inport  Port=8
  landed : Inport  Port=9
  Abs : Abs
  Abs1 : Abs
  Abs2 : Abs
  Add : Sum
  Add1 : Sum
  Add2 : Sum
  Compare To Zero : simulink/Logic and Bit Operations/Compare To Zero  relop=>  OutDataTypeStr=boolean
  Compare To Zero1 : simulink/Logic and Bit Operations/Compare To Zero  relop===  OutDataTypeStr=boolean
  Constant : Constant  Value=1e9
  Data Type Conversion : DataTypeConversion  OutDataTypeStr=double
  Data Type Conversion1 : DataTypeConversion  OutDataTypeStr=double
  Data Type Conversion2 : DataTypeConversion  OutDataTypeStr=double
  Data Type Conversion3 : DataTypeConversion  OutDataTypeStr=uint8
  Divide : Product  Inputs=*/
  Divide1 : Product  Inputs=*/
  Divide2 : Product  Inputs=*/
  Don't Fire : Constant  Value=0
  Force to Maximum Torque Authority With Biprop On : Constant  Value=300
  Gain : Gain  Gain=cac_coarse_desired_thrust_gain
  Half milliseconds of Available Thrusters at 100 ms per axis : Constant  Value=300
  "Half milliseconds of Available Thrusters at 100 ms per axis " : Constant  Value=300
  Half milliseconds of Available Thrusters at 100 ms per axis 1 : Constant  Value=300
  Half milliseconds of Available Thrusters at 100 ms per axis1 : Constant  Value=300
  High end : Constant  Value=100
  Inner Saturation Based on Mass and Extra T/W to Take Off : Saturate  UpperLimit=emp_initial_mass*gal_grav_surface_topo*cac_max_thrust_to_weight_ratio*10  LowerLimit=0
  Inner Saturation Based on Mass and Max T/W : Saturate  UpperLimit=emp_initial_mass*gal_grav_surface_topo*cac_max_thrust_to_weight_ratio  LowerLimit=0
  Logical Operator : Logic  Operator=OR  AllPortsSameDT=off  OutDataTypeStr=boolean
  Logical Operator1 : Logic  Operator=NOT  AllPortsSameDT=off  OutDataTypeStr=boolean
  Logical Operator{2,7,9..12} (6 alike) : Logic  AllPortsSameDT=off  OutDataTypeStr=boolean
  Logical Operator8 : Logic  Operator=OR  Inputs=3  AllPortsSameDT=off  OutDataTypeStr=boolean
  Low end : Constant  Value=0
  MATLAB Function : MATLAB Function  TreatAsAtomicUnit=on
  Max 100 ms : Saturate  UpperLimit=100  LowerLimit=0
  Max Mid Range10 : Constant  Value=0
  Max Mid Range2 : Constant  Value=100
  Max Mid Range3 : Constant  Value=cac_acs_minimum_coarse_thruster_ontime
  Max Mid Range5 : Constant  Value=cac_acs_minimum_coarse_thruster_ontime
  Max Mid Range6 : Constant  Value=100
  Max Mid Range9 : Constant  Value=cac_acs_minimum_coarse_thruster_ontime/2
  Min  Mid Range1 : Constant  Value=cac_acs_minimum_coarse_thruster_ontime
  Min  Mid Range{2..3,6,8} (4 alike) : Constant  Value=100-cac_acs_minimum_coarse_thruster_ontime
  Min  Mid Range4 : Constant  Value=cac_acs_minimum_coarse_thruster_ontime
  Min  Mid Range5 : Constant  Value=100-cac_acs_minimum_coarse_thruster_ontime/2
  Min  Mid Range7 : Constant  Value=100-cac_acs_minimum_coarse_thruster_ontime/2
  Min  Mid Range9 : Constant  Value=cac_acs_minimum_coarse_thruster_ontime
  Outer Saturation Based on Total Thrust Capability : Saturate  UpperLimit=cac_saturation_axial_force  LowerLimit=0
  Product{,1..5} (6 alike) : Product
  Relational Operator{,1,28,30,32,34,36} (7 alike) : RelationalOperator  Operator=>  OutDataTypeStr=boolean
  Relational Operator{24..25,29,31,33,35} (6 alike) : RelationalOperator  OutDataTypeStr=boolean
  Relational Operator26 : RelationalOperator  Operator===  OutDataTypeStr=boolean
  Relational Operator27 : RelationalOperator  Operator===  OutDataTypeStr=boolean
  Sign : Signum
  Sign1 : Signum
  Sign2 : Signum
  Subtract{,2..4} (4 alike) : Sum  Inputs=+-
  Subtract1 : Sum  Inputs=-+
  Subtract5 : Sum  Inputs=-+
  Switch{,1..13} (14 alike) : Switch  Criteria=u2 ~= 0
  Terminator{1..18} (18 alike) : Terminator
  Time Gain : Gain  Gain=cac_acs_time_gain_x
  Time Gain3 : Gain  Gain=cac_acs_time_gain_y
  Time Gain4 : Gain  Gain=cac_acs_time_gain_z
  Total milliseconds of Available Thrusters at 100 ms per axis : Constant  Value=600
  "Total milliseconds of Available Thrusters at 100 ms per axis " : Constant  Value=600
  "Total milliseconds of Available Thrusters at 100 ms per axis  " : Constant  Value=600
  cnt_rotx_deadband_minus1 : Constant  Value=cac_coarse_thruster_trq_x
  cnt_rotx_deadband_minus2 : Constant  Value=cac_coarse_thruster_trq_y
  cnt_rotx_deadband_minus3 : Constant  Value=cac_coarse_thruster_trq_z
  landed1 : InportShadow  Port=9
  "minor frame time Convert to Thrust-msec " : Constant  Value=100
  t_setting_roty_plus1 : Constant  Value=cac_thruster_alloc_pad_coarse_y_tq_full_on
  t_setting_roty_plus10 : Constant  Value=cac_thr_control
  t_setting_roty_plus11 : Constant  Value=cac_trq_control
  t_setting_roty_plus12 : Constant  Value=cac_coarse_thruster_trq_y
  t_setting_roty_plus13 : Constant  Value=cac_coarse_thruster_trq_z
  t_setting_roty_plus2 : Constant  Value=cac_thruster_alloc_pad_coarse_x_tq_variable
  t_setting_roty_plus3 : Constant  Value=cac_thruster_alloc_pad_coarse_y_tq_variable
  t_setting_roty_plus4 : Constant  Value=cac_total_trq_axial_force_matx
  t_setting_roty_plus5 : Constant  Value=cac_saturation_axial_force
  t_setting_roty_plus6 : Constant  Value=cac_num_variable
  t_setting_roty_plus7 : Constant  Value=cac_thruster_alloc_pad_coarse_x_tq_full_on
  t_setting_roty_plus8 : Constant  Value=cac_coarse_thruster_trq_x
  t_setting_roty_plus9 : Constant  Value=cac_coarse_thruster_force
  time_settings : Outport
  wires:
  MATLAB Function/18(torq_axial_cmd) -> Terminator17/1
  MATLAB Function/14(delta_trq_y) -> Terminator16/1
  MATLAB Function/12(delta_thr_y) -> Terminator11/1
  MATLAB Function/10(imax_y) -> Terminator9/1
  Gain/1 -> Inner Saturation Based on Mass and Max T/W/1, Compare To Zero1/1, Inner Saturation Based on Mass and Extra T/W to Take Off/1
  Abs1/1 -> Add/2, Relational Operator1/2, [y_torque_time_cmd], Divide1/1
  Abs/1 -> Divide/1, Add/1, [x_torque_time_cmd], Relational Operator1/1
  Switch1/1 -> MATLAB Function/7(x_sorted_thrust_cmd)
  MATLAB Function/13(delta_trq_x) -> Terminator12/1
  MATLAB Function/17(time_axial_cmd) -> Terminator15/1
  MATLAB Function/5(dist_thrust_y) -> Terminator4/1
  MATLAB Function/3(max_offset_y) -> Terminator2/1
  MATLAB Function/4(dist_thrust_x) -> Terminator3/1
  MATLAB Function/7(radius_minus_distance_x) -> Terminator6/1
  MATLAB Function/9(imax_x) -> Terminator8/1
  MATLAB Function/6(zone_radius) -> Terminator5/1
  MATLAB Function/8(radius_minus_distance_y) -> Terminator7/1
  MATLAB Function/15(coarse_tq_full_on_x) -> Terminator13/1
  MATLAB Function/11(delta_thr_x) -> Terminator10/1
  MATLAB Function/16(coarse_tq_full_on_y) -> Terminator14/1
  MATLAB Function/19(cac_trq_axial_force_pinv_reduced_matx) -> Terminator18/1
  MATLAB Function/2(max_offset_x) -> Terminator1/1
  desired_thrust_in/1 -> Gain/1
  landed1/1 -> Switch11/2
  Inner Saturation Based on Mass and Extra T/W to Take Off/1 -> Switch11/3
  Inner Saturation Based on Mass and Max T/W/1 -> Switch11/1
  Switch11/1 -> Outer Saturation Based on Total Thrust Capability/1
  Switch/1 -> [range_limited_ontime]
  landed/1 -> Logical Operator1/1
  Logical Operator2/1 -> Logical Operator/2
  Compare To Zero1/1 -> Logical Operator2/2
  Logical Operator1/1 -> Logical Operator2/1
  Logical Operator/1 -> Switch6/2
  Compare To Zero/1 -> Logical Operator/1
  Product3/1 -> Switch6/3
  Force to Maximum Torque Authority With Biprop On/1 -> Switch6/1
  Outer Saturation Based on Total Thrust Capability/1 -> Divide2/1, [desired_thrust_time_saturated]
  biprop_cmd_on1/1 -> Compare To Zero/1
  Max 100 ms/1 -> [time_acs_axial_cmd]
  Time Gain3/1 -> Product1/1
  [desired_thrust_time_saturated] -> MATLAB Function/9(desired_thrust_saturated)
  [time_acs_axial_cmd] -> Switch8/1, Relational Operator36/1, Relational Operator35/2, Switch12/3, Relational Operator33/2, Relational Operator34/1, Relational Operator30/1, Relational Operator29/2, Relational Operator28/1, Relational Operator31/2, Relational Operator32/1
  Switch7/1 -> Data Type Conversion3/1
  Switch5/1 -> [y_torque_ontime_y_gt_x]
  Switch4/1 -> [x_torque_ontime_x_gt_y]
  Subtract5/1 -> Switch5/3
  Add2/1 -> Switch5/1
  [thrust_gt_600] -> Switch5/2
  Half milliseconds of Available Thrusters at 100 ms per axis1/1 -> Add2/1
  Product5/1 -> Subtract5/1, Add2/2
  Half milliseconds of Available Thrusters at 100 ms per axis 1/1 -> Subtract5/2
  Subtract1/1 -> Switch4/3
  Add1/1 -> Switch4/1
  [thrust_gt_600] -> Switch4/2
  [range_limited_ontime] -> Product4/2
  [y_frac] -> Product4/1
  [range_limited_ontime] -> Product5/2
  [x_frac] -> Product5/1
  Half milliseconds of Available Thrusters at 100 ms per axis/1 -> Add1/1
  Product4/1 -> Add1/2, Subtract1/1
  "Half milliseconds of Available Thrusters at 100 ms per axis "/1 -> Subtract1/2
  Time Gain4/1 -> Product2/1
  Time Gain/1 -> Product/1
  t_setting_roty_plus3/1 -> MATLAB Function/15(cac_thruster_alloc_pad_coarse_y_tq_variable)
  t_setting_roty_plus4/1 -> MATLAB Function/17(cac_total_trq_axial_force_matx)
  t_setting_roty_plus12/1 -> MATLAB Function/19(cac_coarse_thruster_trq_y)
  t_setting_roty_plus7/1 -> MATLAB Function/12(cac_thruster_alloc_pad_coarse_x_tq_full_on)
  t_setting_roty_plus10/1 -> MATLAB Function/11(cac_thr_control)
  t_setting_roty_plus6/1 -> MATLAB Function/16(cac_num_variable)
  t_setting_roty_plus5/1 -> MATLAB Function/21(cac_saturation_axial_force)
  t_setting_roty_plus13/1 -> MATLAB Function/20(cac_coarse_thruster_trq_z)
  t_setting_roty_plus2/1 -> MATLAB Function/14(cac_thruster_alloc_pad_coarse_x_tq_variable)
  t_setting_roty_plus8/1 -> MATLAB Function/18(cac_coarse_thruster_trq_x)
  t_setting_roty_plus11/1 -> MATLAB Function/10(cac_trq_control)
  t_setting_roty_plus1/1 -> MATLAB Function/13(cac_thruster_alloc_pad_coarse_y_tq_full_on)
  [z_torque_time_cmd] -> MATLAB Function/6(z_torque_time_cmd)
  [z_torque_sign_cmd] -> MATLAB Function/3(z_torque_sign_cmd)
  MATLAB Function/1(time_cmd_total) -> Max 100 ms/1
  Divide/1 -> [x_frac]
  Switch3/1 -> Divide/2, Divide1/2
  Constant/1 -> Switch3/3
  Add/1 -> Switch3/2, Switch3/1
  Switch6/1 -> Subtract/1, Relational Operator/1, Subtract2/2, Subtract4/1, Subtract3/1
  [x_torque_sign_cmd] -> MATLAB Function/1(x_torque_sign_cmd)
  Abs2/1 -> [z_torque_time_cmd]
  Product2/1 -> Abs2/1
  Switch2/1 -> MATLAB Function/8(y_sorted_thrust_cmd)
  [y_torque_sign_cmd] -> MATLAB Function/2(y_torque_sign_cmd)
  [x_torque_time_cmd] -> MATLAB Function/4(x_torque_time_cmd)
  [y_torque_time_cmd] -> MATLAB Function/5(y_torque_time_cmd)
  Data Type Conversion/1 -> [x_torque_sign_cmd]
  Data Type Conversion1/1 -> [y_torque_sign_cmd]
  Data Type Conversion2/1 -> [z_torque_sign_cmd]
  trq_z/1 -> Sign2/1
  Sign2/1 -> Data Type Conversion2/1
  trq_y/1 -> Sign1/1
  Sign1/1 -> Data Type Conversion1/1
  "trq_x "/1 -> Sign/1
  Sign/1 -> Data Type Conversion/1
  [x_torque_ontime_x_gt_y] -> Switch1/1
  [x_torque_ontime_y_gt_x] -> Switch1/3
  [y_torque_ontime_y_gt_x] -> Switch2/3
  [y_torque_ontime_x_gt_y] -> Switch2/1
  Relational Operator1/1 -> Switch2/2, Switch1/2
  Subtract4/1 -> [x_torque_ontime_y_gt_x]
  [y_torque_ontime_y_gt_x] -> Subtract4/2
  Subtract3/1 -> [y_torque_ontime_x_gt_y]
  [x_torque_ontime_x_gt_y] -> Subtract3/2
  Divide1/1 -> [y_frac]
  Subtract2/1 -> Switch/3
  "Total milliseconds of Available Thrusters at 100 ms per axis  "/1 -> Subtract2/1
  Subtract/1 -> Switch/1
  "Total milliseconds of Available Thrusters at 100 ms per axis "/1 -> Subtract/2
  Relational Operator/1 -> Switch/2, [thrust_gt_600]
  Total milliseconds of Available Thrusters at 100 ms per axis/1 -> Relational Operator/2
  Divide2/1 -> Product3/1
  t_setting_roty_plus9/1 -> Divide2/2
  "minor frame time Convert to Thrust-msec "/1 -> Product3/2
  Product1/1 -> Abs1/1
  Product/1 -> Abs/1
  cnt_rotx_deadband_minus3/1 -> Product2/2
  cnt_rotx_deadband_minus2/1 -> Product1/2
  time_z/1 -> Time Gain4/1
  time_y/1 -> Time Gain3/1
  time_x/1 -> Time Gain/1
  cnt_rotx_deadband_minus1/1 -> Product/2
  Max Mid Range10/1 -> Switch9/3
  Switch12/1 -> Switch13/3
  Switch13/1 -> Switch8/3
  Min  Mid Range2/1 -> Switch13/1
  Logical Operator12/1 -> Switch13/2
  Relational Operator36/1 -> Logical Operator12/2
  Relational Operator35/1 -> Logical Operator12/1
  Max Mid Range2/1 -> Switch12/1
  Logical Operator11/1 -> Switch12/2
  Relational Operator34/1 -> Logical Operator11/2
  Relational Operator33/1 -> Logical Operator11/1
  Min  Mid Range8/1 -> Relational Operator36/2
  Min  Mid Range7/1 -> Relational Operator35/1
  Min  Mid Range5/1 -> Relational Operator34/2
  Max Mid Range6/1 -> Relational Operator33/1
  Switch8/1 -> Switch10/1
  Relational Operator28/1 -> Switch10/2
  Min  Mid Range4/1 -> Relational Operator28/2
  Switch10/1 -> Relational Operator26/1, Relational Operator27/1, Switch7/1, Relational Operator24/2, Relational Operator25/1
  Switch9/1 -> Switch10/3
  Logical Operator9/1 -> Switch8/2
  Min  Mid Range9/1 -> Switch9/1
  Logical Operator10/1 -> Switch9/2
  Relational Operator32/1 -> Logical Operator10/2
  Relational Operator31/1 -> Logical Operator10/1
  Max Mid Range9/1 -> Relational Operator32/2
  Max Mid Range3/1 -> Relational Operator31/1
  Relational Operator30/1 -> Logical Operator9/2
  Relational Operator29/1 -> Logical Operator9/1
  Min  Mid Range1/1 -> Relational Operator30/2
  Min  Mid Range6/1 -> Relational Operator29/1
  Don't Fire/1 -> Switch7/3
  Logical Operator8/1 -> Switch7/2
  Low end/1 -> Relational Operator26/2
  Relational Operator26/1 -> Logical Operator8/3
  Logical Operator7/1 -> Logical Operator8/2
  Relational Operator27/1 -> Logical Operator8/1
  High end/1 -> Relational Operator27/2
  Max Mid Range5/1 -> Relational Operator25/2
  Min  Mid Range3/1 -> Relational Operator24/1
  Relational Operator25/1 -> Logical Operator7/2
  Relational Operator24/1 -> Logical Operator7/1
  Data Type Conversion3/1 -> time_settings/1
